simulink model "Example_1_Simu"  (R2023a)
settings: Solver=ode45  StartTime=0.0  StopTime=t_end  FixedStep=1e-6  RelTol=relTol  AbsTol=absTol
undefined symbols (not defined in the file or in its folder): Ag, gamma, InitialOffset, omegag, RayCoe, X, Y, Z
libraries: slrealtimeloglib x26, nesl_utility x19, sm_lib x9, OxDynamicsContact x4, sharedtransform x1
settings Model: Creator=sagat  LastModifiedBy=sagat
settings SolverCC: ConcurrentTasks=on
settings DataIOCC: Decimation=50  FinalStateName=xInitial  InitialState=xinitial  SaveOperatingPoint=on  SaveState=on  ReturnWorkspaceOutputs=off  LoggingToFile=on  LoggingFileName=D:\CODING\Simscape\FinalInvestigation\UniformDamping\LongBeam\ColumnResults
settings OptimizationCC: BlockReduction=off  DefaultParameterBehavior=Inlined  OptimizeBlockIOStorage=off  BufferReuse=off  OptimizeDataStoreBuffers=off  BusAssignmentInplaceUpdate=off
settings DebuggingCC: UnconnectedInputMsg=warning  UnconnectedOutputMsg=warning  UnconnectedLineMsg=warning  SFUnexpectedBacktrackingDiag=warning  SFNoUnconditionalDefaultTransitionDiag=warning
settings HardwareCC: TargetBitPerPointer=64  TargetBitPerSizeT=64  TargetBitPerPtrDiffT=64  TargetLongLongMode=on  TargetIntDivRoundTo=Zero  TargetEndianess=LittleEndian  TargetWordSize=64  TargetHWDeviceType=MATLAB Host  ProdEqTarget=off
settings ModelReferenceCC: EnableRefExpFcnMdlSchedulingChecks=on
settings RTWCC: Description=Rapid Simulation Target  SystemTargetFile=rsim.tlc  GenCodeOnly=on  TemplateMakefile=rsim_default_tmf  GenerateReport=on  BuildConfiguration=Debug  LaunchReport=on  DLArmComputeVersion=19.05
settings CodeAppCC: ForceParamTrailComments=on  MATLABSourceComments=on  EnableCustomComments=on
settings RSimTargetCC: TargetLangStandard=C99 (ISO)  OptimizeReductions=off
settings ExplorerConfigSet: SimMechanicsOpenEditorOnUpdate=off

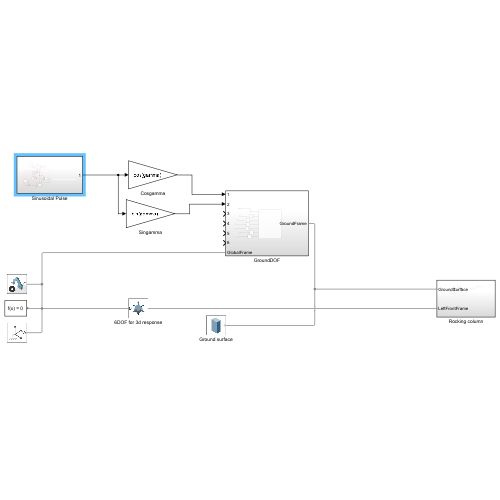
[thumbnail: Simulink's stored preview of the top-level diagram]
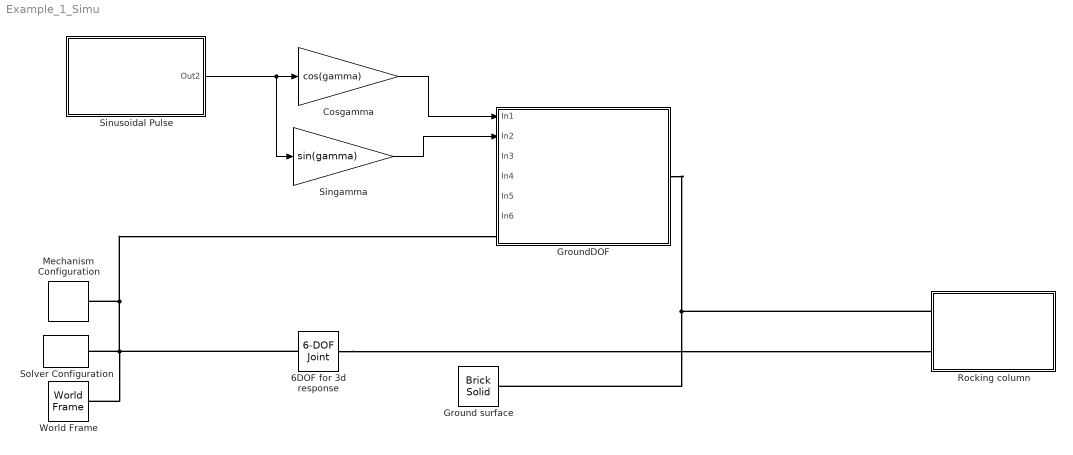
== system Example_1_Simu ==
  6DOF for 3d response : sm_lib/Joints/6-DOF Joint  JointMode=Normal  SenseConstraintForce=off  SenseConstraintForceX=off  SenseConstraintForceY=off  SenseConstraintForceZ=off  SenseConstraintTorque=off  SenseConstraintTorqueX=off  SenseConstraintTorqueY=off  SenseConstraintTorqueZ=off  SenseTotalForce=off  SenseTotalForceX=off  SenseTotalForceY=off  SenseTotalForceZ=off  SenseTotalTorque=off  SenseTotalTorqueX=off  SenseTotalTorqueY=off  SenseTotalTorqueZ=off  CompositeWrenchDir=FollowerOnBase  CompositeWrenchFrame=BaseFrame  PxEquilibriumPosition=0  PxEquilibriumPositionUnits=m  PxSpringStiffness=0  PxSpringStiffnessUnits=N/m  PxDampingCoefficient=0  PxDampingCoefficientUnits=N/(m/s)  PxTorqueActuationMode=NoTorque  PxMotionActuationMode=ComputedMotion  PxSensePosition=off  PxSenseVelocity=off  PxSenseAcceleration=off  PxSenseTorqueForce=off  PxSenseLowerLimitTorqueForce=off  PxSenseUpperLimitTorqueForce=off  PxLowerLimitSpecify=off  PxLowerLimitBound=-1  PxLowerLimitBoundUnits=m  PxLowerLimitStiffness=1e6  PxLowerLimitStiffnessUnits=N/m  PxLowerLimitDamping=1e3  PxLowerLimitDampingUnits=N/(m/s)  PxLowerLimitTransitionRegionWidth=1e-4  PxLowerLimitTransitionRegionWidthUnits=m  PxUpperLimitSpecify=off  PxUpperLimitBound=1  PxUpperLimitBoundUnits=m  PxUpperLimitStiffness=1e6  PxUpperLimitStiffnessUnits=N/m  PxUpperLimitDamping=1e3  PxUpperLimitDampingUnits=N/(m/s)  PxUpperLimitTransitionRegionWidth=1e-4  PxUpperLimitTransitionRegionWidthUnits=m  PxPositionTargetSpecify=on  PxPositionTargetPriority=High  PxPositionTargetValue=0  PxPositionTargetValueUnits=m  PxVelocityTargetSpecify=on  PxVelocityTargetPriority=High  PxVelocityTargetValue=0  PxVelocityTargetValueUnits=m/s  PyEquilibriumPosition=0  PyEquilibriumPositionUnits=m  PySpringStiffness=0  PySpringStiffnessUnits=N/m  PyDampingCoefficient=0  PyDampingCoefficientUnits=N/(m/s)  PyTorqueActuationMode=NoTorque  PyMotionActuationMode=ComputedMotion  PySensePosition=off  PySenseVelocity=off  PySenseAcceleration=off  PySenseTorqueForce=off  PySenseLowerLimitTorqueForce=off  PySenseUpperLimitTorqueForce=off  PyLowerLimitSpecify=off  PyLowerLimitBound=-1  PyLowerLimitBoundUnits=m  PyLowerLimitStiffness=1e6  PyLowerLimitStiffnessUnits=N/m  PyLowerLimitDamping=1e3  PyLowerLimitDampingUnits=N/(m/s)  PyLowerLimitTransitionRegionWidth=1e-4  PyLowerLimitTransitionRegionWidthUnits=m  PyUpperLimitSpecify=off  PyUpperLimitBound=1  PyUpperLimitBoundUnits=m  PyUpperLimitStiffness=1e6  PyUpperLimitStiffnessUnits=N/m  PyUpperLimitDamping=1e3  PyUpperLimitDampingUnits=N/(m/s)  PyUpperLimitTransitionRegionWidth=1e-4  PyUpperLimitTransitionRegionWidthUnits=m  PyPositionTargetSpecify=on  PyPositionTargetPriority=High  PyPositionTargetValue=0  PyPositionTargetValueUnits=m  PyVelocityTargetSpecify=on  PyVelocityTargetPriority=High  PyVelocityTargetValue=0  PyVelocityTargetValueUnits=m/s  PzEquilibriumPosition=0  PzEquilibriumPositionUnits=m  PzSpringStiffness=0  PzSpringStiffnessUnits=N/m  PzDampingCoefficient=0  PzDampingCoefficientUnits=N/(m/s)  PzTorqueActuationMode=NoTorque  PzMotionActuationMode=ComputedMotion  PzSensePosition=off  PzSenseVelocity=off  PzSenseAcceleration=off  PzSenseTorqueForce=off  PzSenseLowerLimitTorqueForce=off  PzSenseUpperLimitTorqueForce=off  PzLowerLimitSpecify=off  PzLowerLimitBound=-1  PzLowerLimitBoundUnits=m  PzLowerLimitStiffness=1e6  PzLowerLimitStiffnessUnits=N/m  PzLowerLimitDamping=1e3  PzLowerLimitDampingUnits=N/(m/s)  PzLowerLimitTransitionRegionWidth=1e-4  PzLowerLimitTransitionRegionWidthUnits=m  PzUpperLimitSpecify=off  PzUpperLimitBound=1  PzUpperLimitBoundUnits=m  PzUpperLimitStiffness=1e6  PzUpperLimitStiffnessUnits=N/m  PzUpperLimitDamping=1e3  PzUpperLimitDampingUnits=N/(m/s)  PzUpperLimitTransitionRegionWidth=1e-4  PzUpperLimitTransitionRegionWidthUnits=m  PzPositionTargetSpecify=on  PzPositionTargetPriority=High  PzPositionTargetValue=zc  PzPositionTargetValueUnits=m  PzVelocityTargetSpecify=on  PzVelocityTargetPriority=High  PzVelocityTargetValue=0  PzVelocityTargetValueUnits=m/s  SphEqPosRotationMethod=None  SphEqPosRotationAngleUnits=rad  SphEqPosRotationStandardAxis=-Y  SphEqPosRotationAngle=alphacg  SphEqPosRotationArbitraryAxis=[0 0 1]  SphEqPosFollAlignAxisA=+X  SphEqPosBaseAlignAxisA=+Y  SphEqPosFollAlignAxisB=+Y  SphEqPosBaseAlignAxisB=+Z  SphEqPosRotationSequenceAxes=FollowerAxes  SphEqPosRotationSequence=XYX  SphEqPosRotationSequenceAngles=[0 0 0]  SphEqPosRotationSequenceAnglesUnits=deg  SphEqPosRotationMatrix=[1 0 0; 0 1 0; 0 0 1]  SphEqPosQuaternion=[1 0 0 0]  SphSpringStiffness=0  SphSpringStiffnessUnits=N*m/rad  SphDampingCoefficient=0  SphDampingCoefficientUnits=N*m/(rad/s)  SphActuateTorqueX=off  SphActuateTorqueY=off  SphActuateTorqueZ=off  SphActuateTorque=off  SphTorqueActuationMode=NoTorque  SphMotionActuationMode=ComputedMotion  SphActuationFrame=BaseFrame  SphSensePosition=off  SphSenseVelocityX=off  SphSenseVelocityY=off  SphSenseVelocityZ=off  SphSenseVelocity=off  SphSenseAccelerationX=off  SphSenseAccelerationY=off  SphSenseAccelerationZ=off  SphSenseAcceleration=off  SphSenseTorqueX=off  SphSenseTorqueY=off  SphSenseTorqueZ=off  SphSenseTorqueForce=off  SphSenseLowerLimitTorqueMag=off  SphSenseUpperLimitTorqueMag=off  SphSensingFrame=BaseFrame  SphLowerLimitSpecify=off  SphLowerLimitBound=15  SphLowerLimitBoundUnits=deg  SphLowerLimitStiffness=1e4  SphLowerLimitStiffnessUnits=N*m/deg  SphLowerLimitDamping=10  SphLowerLimitDampingUnits=N*m/(deg/s)  SphLowerLimitTransitionRegionWidth=0.1  SphLowerLimitTransitionRegionWidthUnits=deg  SphUpperLimitSpecify=off  SphUpperLimitBound=45  SphUpperLimitBoundUnits=deg  SphUpperLimitStiffness=1e4  SphUpperLimitStiffnessUnits=N*m/deg  SphUpperLimitDamping=10  SphUpperLimitDampingUnits=N*m/(deg/s)  SphUpperLimitTransitionRegionWidth=0.1  SphUpperLimitTransitionRegionWidthUnits=deg  SphPositionTargetRotationMethod=StandardAxis  SphPositionTargetRotationAngleUnits=rad  SphPositionTargetRotationStandardAxis=-Y  SphPositionTargetRotationAngle=initialRotation  SphPositionTargetRotationArbitraryAxis=[0 0 1]  SphPositionTargetFollAlignAxisA=+X  SphPositionTargetBaseAlignAxisA=+Y  SphPositionTargetFollAlignAxisB=+Y  SphPositionTargetBaseAlignAxisB=+Z  SphPositionTargetRotationSequenceAxes=FollowerAxes  SphPositionTargetRotationSequence=XYX  SphPositionTargetRotationSequenceAngles=[0 0 0]  SphPositionTargetRotationSequenceAnglesUnits=deg  SphPositionTargetRotationMatrix=[1 0 0; 0 1 0; 0 0 1]  SphPositionTargetQuaternion=[1 0 0 0]  SphPositionTargetSpecify=on  SphPositionTargetPriority=High  SphVelocityTargetValue=[0 0 0]  SphVelocityTargetValueUnits=deg/s  SphVelocityTargetSpecify=on  SphVelocityTargetPriority=High  SphVelocityTargetInFollowerFrame=on
  Cosgamma : Gain  Gain=cos(gamma)
  Ground surface : sm_lib/Body Elements/Brick Solid  GraphicAmbientColor=[0.15 0.15 0.15 1.0]  BasedOnType=Density  BrickDimensions=[5 5 0.01]  BrickDimensionsUnits=m  CenterOfMass=[0 0 0]  CenterOfMassUnits=m  GraphicDiffuseColor=[0.5 0.5 0.5]  Density=1  DensityUnits=kg/m^3  DoExposeReferenceFrame=on  GraphicEmissiveColor=[0.0 0.0 0.0 1.0]  ExportEntireGeometry=off  SerializedFrames=<Frames/>  MarkerShape=Sphere  MarkerSize=10  GraphicType=FromGeometry  InertiaType=CalculateFromGeometry  Mass=1  MassUnits=kg  MomentsOfInertia=[1 1 1]  MomentsOfInertiaUnits=kg*m^2  GraphicOpacity=1.0  ProductsOfInertia=[0 0 0]  ProductsOfInertiaUnits=kg*m^2  GraphicShininess=75  GraphicSpecularColor=[0.5 0.5 0.5 1.0]  GraphicVisPropType=SimpleVisualProperties
  GroundDOF : Subsystem
  Mechanism Configuration : sm_lib/Utilities/Mechanism Configuration  UniformGravity=Constant  GravityVector=[0 0 -9.80665]  GravityVectorUnits=m/s^2  LinearizationDelta=0.001  JointModeTransitionNonlinearIterations=2
  Rocking column : Subsystem
  Singamma : Gain  Gain=sin(gamma)
  Sinusoidal Pulse : Subsystem
  Solver Configuration : nesl_utility/Solver Configuration  PhysicalDomain=network_engine_domain  SubClassName=solver  LeftPortType=input  RightPortType=generic  Tones=[]  Harmonics=[]  SimulateNoise=off  Profile=off  UseLocalSampling=off  EnableSwitchedLinearOptims=on  FrequencyDomain=off  UseCCode=off  RelTol=0.001  AbsTol=1e-06  MinStep=1e-09  ToWorkspace=off  RevertToSquareIcSolve=off  NumHomotopyIterations=100  PhasorMode=off  PhasorModeNumHarmonics=1  ConsistencySolver=NEWTON_FTOL  IndexReductionMethod=DerivativeReplacement  DoDC=off  ResidualTolerance=1e-09  ConsistencyTolSource=GLOBAL  ConsistencyAbsTol=0.001  ConsistencyRelTol=0.001  ConsistencyTolFactor=0.001  UseLocalSolver=off  LocalSolverChoice=NE_BACKWARD_EULER_ADVANCER  ResolveIndetEquations=on  FunctionEvalNumThread=1  LocalSolverSampleTime=0.001  DoFixedCost=off  MaxNonlinIter=3  MaxModeIter=2  ComputeImpulses=off  ImpulseIterations=2  LinearAlgebra=auto  LinearAlgebraNumThread=0  EquationFormulation=NE_TIME_EF  DelaysMemoryBudget=1024  AutomaticFiltering=on  FilteringTimeConstant=0.001  PartitionStorageMethod=AS_NEEDED  PartitionMemoryBudget=1024  PartitionMethod=ROBUST
  World Frame : sm_lib/Frames and Transforms/World Frame
  wires:
  Cosgamma/1 -> GroundDOF/1(In1)
  Sinusoidal Pulse/1(Out2) -> Singamma/1, Cosgamma/1
  Singamma/1 -> GroundDOF/2(In2)
  connections:
  World Frame/RConn1 -- GroundDOF/LConn1 -- Mechanism Configuration/RConn1 -- 6DOF for 3d response/LConn1 -- Solver Configuration/RConn1
  6DOF for 3d response/RConn1 -- Rocking column/LConn2
  GroundDOF/RConn1 -- Rocking column/LConn1 -- Ground surface/RConn1

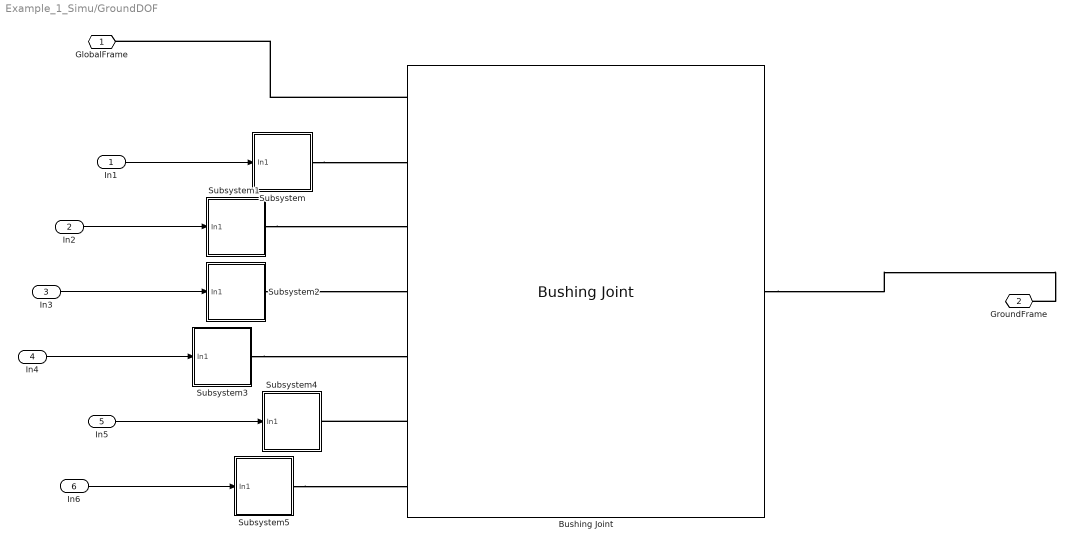
== system Example_1_Simu/GroundDOF ==
  In1 : Inport
  In2 : Inport  Port=2
  In3 : Inport  Port=3
  In4 : Inport  Port=4
  In5 : Inport  Port=5
  In6 : Inport  Port=6
  Bushing Joint : sm_lib/Joints/Bushing Joint  JointMode=Normal  SenseConstraintForce=off  SenseConstraintForceX=off  SenseConstraintForceY=off  SenseConstraintForceZ=off  SenseConstraintTorque=off  SenseConstraintTorqueX=off  SenseConstraintTorqueY=off  SenseConstraintTorqueZ=off  SenseTotalForce=off  SenseTotalForceX=off  SenseTotalForceY=off  SenseTotalForceZ=off  SenseTotalTorque=off  SenseTotalTorqueX=off  SenseTotalTorqueY=off  SenseTotalTorqueZ=off  CompositeWrenchDir=FollowerOnBase  CompositeWrenchFrame=BaseFrame  PxEquilibriumPosition=0  PxEquilibriumPositionUnits=m  PxSpringStiffness=0  PxSpringStiffnessUnits=N/m  PxDampingCoefficient=0  PxDampingCoefficientUnits=N/(m/s)  PxTorqueActuationMode=ComputedTorque  PxMotionActuationMode=InputMotion  PxSensePosition=off  PxSenseVelocity=off  PxSenseAcceleration=off  PxSenseTorqueForce=off  PxSenseLowerLimitTorqueForce=off  PxSenseUpperLimitTorqueForce=off  PxLowerLimitSpecify=off  PxLowerLimitBound=-1  PxLowerLimitBoundUnits=m  PxLowerLimitStiffness=1e6  PxLowerLimitStiffnessUnits=N/m  PxLowerLimitDamping=1e3  PxLowerLimitDampingUnits=N/(m/s)  PxLowerLimitTransitionRegionWidth=1e-4  PxLowerLimitTransitionRegionWidthUnits=m  PxUpperLimitSpecify=off  PxUpperLimitBound=1  PxUpperLimitBoundUnits=m  PxUpperLimitStiffness=1e6  PxUpperLimitStiffnessUnits=N/m  PxUpperLimitDamping=1e3  PxUpperLimitDampingUnits=N/(m/s)  PxUpperLimitTransitionRegionWidth=1e-4  PxUpperLimitTransitionRegionWidthUnits=m  PxPositionTargetSpecify=off  PxPositionTargetPriority=High  PxPositionTargetValue=0  PxPositionTargetValueUnits=m  PxVelocityTargetSpecify=off  PxVelocityTargetPriority=High  PxVelocityTargetValue=0  PxVelocityTargetValueUnits=m/s  PyEquilibriumPosition=0  PyEquilibriumPositionUnits=m  PySpringStiffness=0  PySpringStiffnessUnits=N/m  PyDampingCoefficient=0  PyDampingCoefficientUnits=N/(m/s)  PyTorqueActuationMode=ComputedTorque  PyMotionActuationMode=InputMotion  PySensePosition=off  PySenseVelocity=off  PySenseAcceleration=off  PySenseTorqueForce=off  PySenseLowerLimitTorqueForce=off  PySenseUpperLimitTorqueForce=off  PyLowerLimitSpecify=off  PyLowerLimitBound=-1  PyLowerLimitBoundUnits=m  PyLowerLimitStiffness=1e6  PyLowerLimitStiffnessUnits=N/m  PyLowerLimitDamping=1e3  PyLowerLimitDampingUnits=N/(m/s)  PyLowerLimitTransitionRegionWidth=1e-4  PyLowerLimitTransitionRegionWidthUnits=m  PyUpperLimitSpecify=off  PyUpperLimitBound=1  PyUpperLimitBoundUnits=m  PyUpperLimitStiffness=1e6  PyUpperLimitStiffnessUnits=N/m  PyUpperLimitDamping=1e3  PyUpperLimitDampingUnits=N/(m/s)  PyUpperLimitTransitionRegionWidth=1e-4  PyUpperLimitTransitionRegionWidthUnits=m  PyPositionTargetSpecify=off  PyPositionTargetPriority=High  PyPositionTargetValue=0  PyPositionTargetValueUnits=m  PyVelocityTargetSpecify=off  PyVelocityTargetPriority=High  PyVelocityTargetValue=0  PyVelocityTargetValueUnits=m/s  PzEquilibriumPosition=0  PzEquilibriumPositionUnits=m  PzSpringStiffness=0  PzSpringStiffnessUnits=N/m  PzDampingCoefficient=0  PzDampingCoefficientUnits=N/(m/s)  PzTorqueActuationMode=ComputedTorque  PzMotionActuationMode=InputMotion  PzSensePosition=off  PzSenseVelocity=off  PzSenseAcceleration=off  PzSenseTorqueForce=off  PzSenseLowerLimitTorqueForce=off  PzSenseUpperLimitTorqueForce=off  PzLowerLimitSpecify=off  PzLowerLimitBound=-1  PzLowerLimitBoundUnits=m  PzLowerLimitStiffness=1e6  PzLowerLimitStiffnessUnits=N/m  PzLowerLimitDamping=1e3  PzLowerLimitDampingUnits=N/(m/s)  PzLowerLimitTransitionRegionWidth=1e-4  PzLowerLimitTransitionRegionWidthUnits=m  PzUpperLimitSpecify=off  PzUpperLimitBound=1  PzUpperLimitBoundUnits=m  PzUpperLimitStiffness=1e6  PzUpperLimitStiffnessUnits=N/m  PzUpperLimitDamping=1e3  PzUpperLimitDampingUnits=N/(m/s)  PzUpperLimitTransitionRegionWidth=1e-4  PzUpperLimitTransitionRegionWidthUnits=m  PzPositionTargetSpecify=off  PzPositionTargetPriority=High  PzPositionTargetValue=0  PzPositionTargetValueUnits=m  PzVelocityTargetSpecify=off  PzVelocityTargetPriority=High  PzVelocityTargetValue=0  PzVelocityTargetValueUnits=m/s  RxEquilibriumPosition=0  RxEquilibriumPositionUnits=deg  RxSpringStiffness=0  RxSpringStiffnessUnits=N*m/deg  RxDampingCoefficient=0  RxDampingCoefficientUnits=N*m/(deg/s)  RxTorqueActuationMode=ComputedTorque  RxMotionActuationMode=InputMotion  RxSensePosition=off  RxSenseVelocity=off  RxSenseAcceleration=off  RxSenseTorqueForce=off  RxSenseLowerLimitTorqueForce=off  RxSenseUpperLimitTorqueForce=off  RxLowerLimitSpecify=off  RxLowerLimitBound=-90  RxLowerLimitBoundUnits=deg  RxLowerLimitStiffness=1e4  RxLowerLimitStiffnessUnits=N*m/deg  RxLowerLimitDamping=10  RxLowerLimitDampingUnits=N*m/(deg/s)  RxLowerLimitTransitionRegionWidth=0.1  RxLowerLimitTransitionRegionWidthUnits=deg  RxUpperLimitSpecify=off  RxUpperLimitBound=90  RxUpperLimitBoundUnits=deg  RxUpperLimitStiffness=1e4  RxUpperLimitStiffnessUnits=N*m/deg  RxUpperLimitDamping=10  RxUpperLimitDampingUnits=N*m/(deg/s)  RxUpperLimitTransitionRegionWidth=0.1  RxUpperLimitTransitionRegionWidthUnits=deg  RxPositionTargetSpecify=off  RxPositionTargetPriority=High  RxPositionTargetValue=0  RxPositionTargetValueUnits=deg  RxVelocityTargetSpecify=off  RxVelocityTargetPriority=High  RxVelocityTargetValue=0  RxVelocityTargetValueUnits=deg/s  RyEquilibriumPosition=0  RyEquilibriumPositionUnits=deg  RySpringStiffness=0  RySpringStiffnessUnits=N*m/deg  RyDampingCoefficient=0  RyDampingCoefficientUnits=N*m/(deg/s)  RyTorqueActuationMode=ComputedTorque  RyMotionActuationMode=InputMotion  RySensePosition=off  RySenseVelocity=off  RySenseAcceleration=off  RySenseTorqueForce=off  RySenseLowerLimitTorqueForce=off  RySenseUpperLimitTorqueForce=off  RyLowerLimitSpecify=off  RyLowerLimitBound=-90  RyLowerLimitBoundUnits=deg  RyLowerLimitStiffness=1e4  RyLowerLimitStiffnessUnits=N*m/deg  RyLowerLimitDamping=10  RyLowerLimitDampingUnits=N*m/(deg/s)  RyLowerLimitTransitionRegionWidth=0.1  RyLowerLimitTransitionRegionWidthUnits=deg  RyUpperLimitSpecify=off  RyUpperLimitBound=90  RyUpperLimitBoundUnits=deg  RyUpperLimitStiffness=1e4  RyUpperLimitStiffnessUnits=N*m/deg  RyUpperLimitDamping=10  RyUpperLimitDampingUnits=N*m/(deg/s)  RyUpperLimitTransitionRegionWidth=0.1  RyUpperLimitTransitionRegionWidthUnits=deg  RyPositionTargetSpecify=off  RyPositionTargetPriority=High  RyPositionTargetValue=0  RyPositionTargetValueUnits=deg  RyVelocityTargetSpecify=off  RyVelocityTargetPriority=High  RyVelocityTargetValue=0  RyVelocityTargetValueUnits=deg/s  RzEquilibriumPosition=0  RzEquilibriumPositionUnits=deg  RzSpringStiffness=0  RzSpringStiffnessUnits=N*m/deg  RzDampingCoefficient=0  RzDampingCoefficientUnits=N*m/(deg/s)  RzTorqueActuationMode=ComputedTorque  RzMotionActuationMode=InputMotion  RzSensePosition=off  RzSenseVelocity=off  RzSenseAcceleration=off  RzSenseTorqueForce=off  RzSenseLowerLimitTorqueForce=off  RzSenseUpperLimitTorqueForce=off  RzLowerLimitSpecify=off  RzLowerLimitBound=-90  RzLowerLimitBoundUnits=deg  RzLowerLimitStiffness=1e4  RzLowerLimitStiffnessUnits=N*m/deg  RzLowerLimitDamping=10  RzLowerLimitDampingUnits=N*m/(deg/s)  RzLowerLimitTransitionRegionWidth=0.1  RzLowerLimitTransitionRegionWidthUnits=deg  RzUpperLimitSpecify=off  RzUpperLimitBound=90  RzUpperLimitBoundUnits=deg  RzUpperLimitStiffness=1e4  RzUpperLimitStiffnessUnits=N*m/deg  RzUpperLimitDamping=10  RzUpperLimitDampingUnits=N*m/(deg/s)  RzUpperLimitTransitionRegionWidth=0.1  RzUpperLimitTransitionRegionWidthUnits=deg  RzPositionTargetSpecify=off  RzPositionTargetPriority=High  RzPositionTargetValue=0  RzPositionTargetValueUnits=deg  RzVelocityTargetSpecify=off  RzVelocityTargetPriority=High  RzVelocityTargetValue=0  RzVelocityTargetValueUnits=deg/s
  Subsystem : Subsystem
  Subsystem1 : Subsystem
  Subsystem2 : Subsystem
  Subsystem3 : Subsystem
  Subsystem4 : Subsystem
  Subsystem5 : Subsystem
  GlobalFrame : PMIOPort  Side=Left
  GroundFrame : PMIOPort  Port=2  Side=Right
  wires:
  In1/1 -> Subsystem/1(In1)
  In5/1 -> Subsystem4/1(In1)
  In2/1 -> Subsystem1/1(In1)
  In3/1 -> Subsystem2/1(In1)
  In4/1 -> Subsystem3/1(In1)
  In6/1 -> Subsystem5/1(In1)
  connections:
  Bushing Joint/LConn1 -- GlobalFrame/RConn1
  Subsystem3/RConn1 -- Bushing Joint/LConn5
  Subsystem/RConn1 -- Bushing Joint/LConn2
  Bushing Joint/LConn6 -- Subsystem4/RConn1
  Subsystem2/RConn1 -- Bushing Joint/LConn4
  Subsystem5/RConn1 -- Bushing Joint/LConn7
  Bushing Joint/RConn1 -- GroundFrame/RConn1
  Subsystem1/RConn1 -- Bushing Joint/LConn3

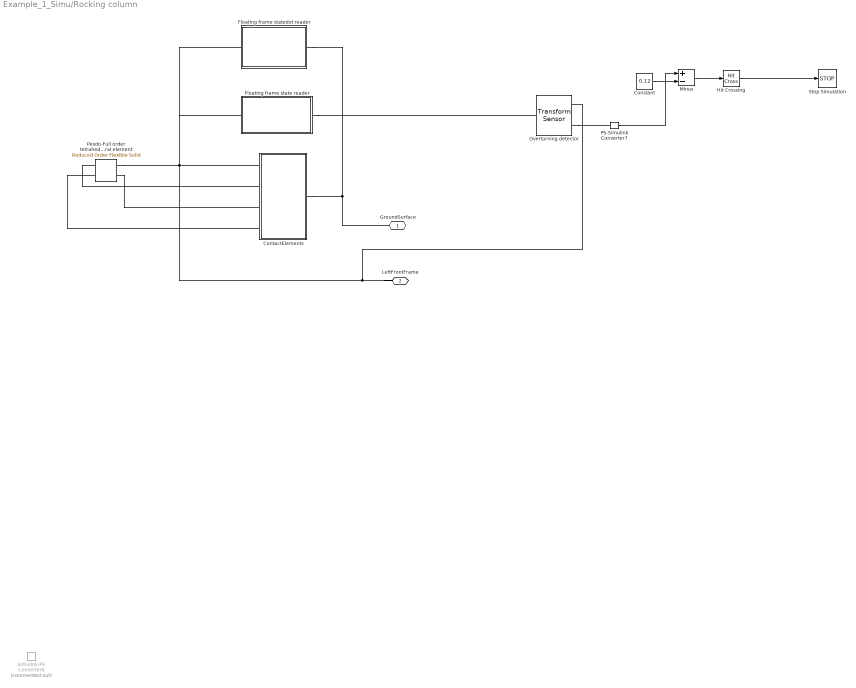
== system Example_1_Simu/Rocking column ==
  Constant : Constant  Value=0.12
  ContactElements : Subsystem
  Floating frame state reader : Subsystem
  Floating frame statedot reader : Subsystem
  Hit Crossing : HitCross
  Minus : Sum  Inputs=+-
  Overturning detector : sm_lib/Frames and Transforms/Transform Sensor  MeasurementFrame=Base  RotationSequence=XYX  SenseAngle=on  SenseAxis=off  SenseQ=off  SenseR=off  SenseRotationSequence=off  SenseOmegaX=off  SenseOmegaY=off  SenseOmegaZ=off  SenseQDot=off  SenseRDot=off  SenseRotationSequenceDot=off  SenseAlphaX=off  SenseAlphaY=off  SenseAlphaZ=off  SenseQDDot=off  SenseRDDot=off  SenseX=off  SenseY=off  SenseZ=off  SenseRad=off  SenseAzim=off  SenseDist=off  SenseInc=off  SenseXDot=off  SenseYDot=off  SenseZDot=off  SenseRadDot=off  SenseAzimDot=off  SenseDistDot=off  SenseIncDot=off  SenseXDDot=off  SenseYDDot=off  SenseZDDot=off  SenseRadDDot=off  SenseAzimDDot=off  SenseDistDDot=off  SenseIncDDot=off
  PS-Simulink Converter7 : nesl_utility/PS-Simulink Converter  PhysicalDomain=network_engine_domain  SubClassName=ps_output  LeftPortType=input  RightPortType=output  PseudoPeriodic=off  Frequencies=[]  VectorFormat=1-D array  Unit=inherit  AffineConversion=off
  Pesdo-Full order tetrahedral element : sm_lib/Body Elements/Flexible Bodies/Reduced Order Flexible Solid  GraphicAmbientColor=[0.15 0.15 0.15 1.0]  GraphicDiffuseColor=[0.5 0.5 0.5]  DampingType=DampingMatrix  GraphicEmissiveColor=[0.0 0.0 0.0 1.0]  GraphicFacetVertexIndices=[]  GeomFileName=D:\CODING\Simscape\ReducedSuperStructure&AxialDeformationInvestigation\WaterTank\Trial2.stl  InterfaceFrameOrientations=[1 0 0 0;1 0 0 0;1 0 0 0;1 0 0 0]  GraphicType=None  MassMatrix=Reduced.M  NumRetainedModes=1  NumberOfInterfaceFrames=4  GraphicOpacity=1.0  GraphicReconstructionMatrix=[]  ReductionType=None  InterfaceFrameOrigins=Reduced.P  GraphicShininess=75  GraphicSpecularColor=[0.5 0.5 0.5 1.0]  StiffnessMatrix=Reduced.K  GeomUnitType=FromUnitSystem  GraphicVertexCoordinates=[]  VisRecursionLimit=3  GraphicVisPropType=SimpleVisualProperties  LengthUnit=m  MassUnit=kg  TimeUnit=s  UnitSystemType=SI  ProportionalDampingAlpha=0  ProportionalDampingBeta=RayCoe(2)  UniformModalDampingRatio=0.05  DampingMatrix=Reduced.C
  Simulink-PS Converter6 : nesl_utility/Simulink-PS Converter  Commented=on  PhysicalDomain=network_engine_domain  SubClassName=ps_input  LeftPortType=input  RightPortType=output  PseudoPeriodic=off  Frequencies=[]  NoiseDistribution=none  NoiseParameters=[]  Unit=1  AffineConversion=off  FilteringAndDerivatives=provide  SimscapeFilterOrder=1  InputFilterTimeConstant=0.001  UdotUserProvided=0
  Stop Simulation : Stop
  GroundSurface : PMIOPort  Side=Left
  LeftFrontFrame : PMIOPort  Port=2  Side=Left
  wires:
  PS-Simulink Converter7/1 -> Minus/1
  Minus/1 -> Hit Crossing/1
  Hit Crossing/1 -> Stop Simulation/1
  Constant/1 -> Minus/2
  connections:
  Pesdo-Full order tetrahedral element/LConn1 -- Floating frame state reader/RConn1 -- Floating frame statedot reader/RConn1 -- ContactElements/LConn1 -- Overturning detector/RConn1 -- LeftFrontFrame/RConn1
  Pesdo-Full order tetrahedral element/RConn1 -- ContactElements/LConn2
  Pesdo-Full order tetrahedral element/LConn2 -- ContactElements/LConn3
  Pesdo-Full order tetrahedral element/RConn2 -- ContactElements/LConn4
  ContactElements/RConn1 -- Floating frame statedot reader/LConn1 -- Floating frame state reader/LConn1 -- Overturning detector/LConn1 -- GroundSurface/RConn1
  Overturning detector/RConn2 -- PS-Simulink Converter7/LConn1

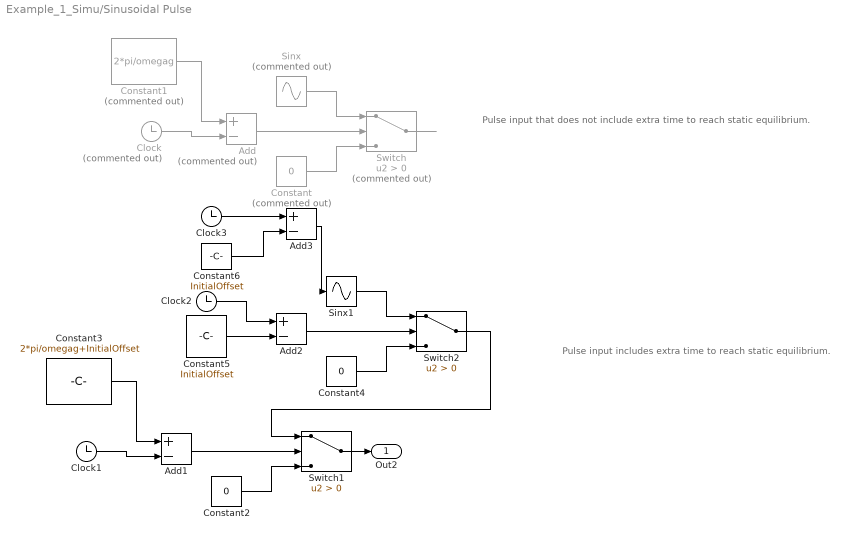
== system Example_1_Simu/Sinusoidal Pulse ==
  note: Pulse input that does not include extra time to reach static equilibrium.
  note: Pulse input includes extra time to reach static equilibrium.
  Add : Sum  Commented=on  Inputs=+-
  Add1 : Sum  Inputs=+-
  Add2 : Sum  Inputs=+-
  Add3 : Sum  Inputs=+-
  Clock : Clock  Commented=on
  Clock1 : Clock
  Clock2 : Clock
  Clock3 : Clock
  Constant : Constant  Commented=on  Value=0
  Constant1 : Constant  Commented=on  Value=2*pi/omegag
  Constant2 : Constant  Value=0
  Constant3 : Constant  Value=2*pi/omegag+InitialOffset
  Constant4 : Constant  Value=0
  Constant5 : Constant  Value=InitialOffset
  Constant6 : Constant  Value=InitialOffset
  Sinx : Sin  Commented=on  Amplitude=Ag  Frequency=omegag  SampleTime=0
  Sinx1 : Sin  TimeSource=Use external signal  Amplitude=Ag  Frequency=omegag  SampleTime=0
  Switch : Switch  Commented=on  Criteria=u2 > Threshold  SaturateOnIntegerOverflow=off  InputSameDT=off
  Switch1 : Switch  Criteria=u2 > Threshold  SaturateOnIntegerOverflow=off  InputSameDT=off
  Switch2 : Switch  Criteria=u2 > Threshold  SaturateOnIntegerOverflow=off  InputSameDT=off
  Out2 : Outport
  wires:
  Clock/1 -> Add/2
  Switch/1 -> ?
  Constant1/1 -> Add/1
  Sinx/1 -> Switch/1
  Constant/1 -> Switch/3
  Add/1 -> Switch/2
  Switch1/1 -> Out2/1
  Clock1/1 -> Add1/2
  Constant2/1 -> Switch1/3
  Add1/1 -> Switch1/2
  Constant3/1 -> Add1/1
  Switch2/1 -> Switch1/1
  Constant4/1 -> Switch2/3
  Add2/1 -> Switch2/2
  Sinx1/1 -> Switch2/1
  Clock2/1 -> Add2/1
  Constant5/1 -> Add2/2
  Clock3/1 -> Add3/1
  Constant6/1 -> Add3/2
  Add3/1 -> Sinx1/1

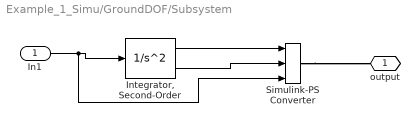
== system Example_1_Simu/GroundDOF/Subsystem ==
  In1 : Inport
  "Integrator, Second-Order" : SecondOrderIntegrator
  Simulink-PS Converter : nesl_utility/Simulink-PS Converter  PhysicalDomain=network_engine_domain  SubClassName=ps_input  LeftPortType=input  RightPortType=output  PseudoPeriodic=off  Frequencies=[]  NoiseDistribution=none  NoiseParameters=[]  Unit=1  AffineConversion=off  FilteringAndDerivatives=provide  SimscapeFilterOrder=1  InputFilterTimeConstant=0.001  UdotUserProvided=2
  output : PMIOPort  Side=Right
  wires:
  "Integrator, Second-Order"/1 -> Simulink-PS Converter/1
  "Integrator, Second-Order"/2 -> Simulink-PS Converter/2
  In1/1 -> "Integrator, Second-Order"/1, Simulink-PS Converter/3
  connections:
  Simulink-PS Converter/RConn1 -- output/RConn1

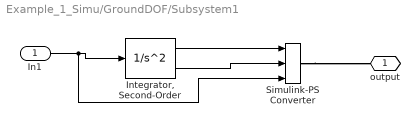
== system Example_1_Simu/GroundDOF/Subsystem1 ==
  In1 : Inport
  "Integrator, Second-Order" : SecondOrderIntegrator
  Simulink-PS Converter : nesl_utility/Simulink-PS Converter  PhysicalDomain=network_engine_domain  SubClassName=ps_input  LeftPortType=input  RightPortType=output  PseudoPeriodic=off  Frequencies=[]  NoiseDistribution=none  NoiseParameters=[]  Unit=1  AffineConversion=off  FilteringAndDerivatives=provide  SimscapeFilterOrder=1  InputFilterTimeConstant=0.001  UdotUserProvided=2
  output : PMIOPort  Side=Right
  wires:
  "Integrator, Second-Order"/1 -> Simulink-PS Converter/1
  "Integrator, Second-Order"/2 -> Simulink-PS Converter/2
  In1/1 -> "Integrator, Second-Order"/1, Simulink-PS Converter/3
  connections:
  Simulink-PS Converter/RConn1 -- output/RConn1

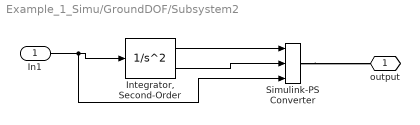
== system Example_1_Simu/GroundDOF/Subsystem2 ==
  In1 : Inport
  "Integrator, Second-Order" : SecondOrderIntegrator
  Simulink-PS Converter : nesl_utility/Simulink-PS Converter  PhysicalDomain=network_engine_domain  SubClassName=ps_input  LeftPortType=input  RightPortType=output  PseudoPeriodic=off  Frequencies=[]  NoiseDistribution=none  NoiseParameters=[]  Unit=1  AffineConversion=off  FilteringAndDerivatives=provide  SimscapeFilterOrder=1  InputFilterTimeConstant=0.001  UdotUserProvided=2
  output : PMIOPort  Side=Right
  wires:
  "Integrator, Second-Order"/1 -> Simulink-PS Converter/1
  "Integrator, Second-Order"/2 -> Simulink-PS Converter/2
  In1/1 -> "Integrator, Second-Order"/1, Simulink-PS Converter/3
  connections:
  Simulink-PS Converter/RConn1 -- output/RConn1

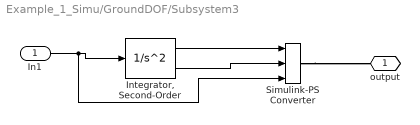
== system Example_1_Simu/GroundDOF/Subsystem3 ==
  In1 : Inport
  "Integrator, Second-Order" : SecondOrderIntegrator
  Simulink-PS Converter : nesl_utility/Simulink-PS Converter  PhysicalDomain=network_engine_domain  SubClassName=ps_input  LeftPortType=input  RightPortType=output  PseudoPeriodic=off  Frequencies=[]  NoiseDistribution=none  NoiseParameters=[]  Unit=1  AffineConversion=off  FilteringAndDerivatives=provide  SimscapeFilterOrder=1  InputFilterTimeConstant=0.001  UdotUserProvided=2
  output : PMIOPort  Side=Right
  wires:
  In1/1 -> Simulink-PS Converter/3, "Integrator, Second-Order"/1
  "Integrator, Second-Order"/2 -> Simulink-PS Converter/2
  "Integrator, Second-Order"/1 -> Simulink-PS Converter/1
  connections:
  Simulink-PS Converter/RConn1 -- output/RConn1

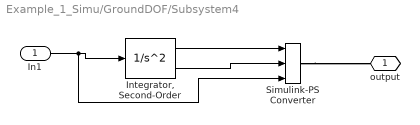
== system Example_1_Simu/GroundDOF/Subsystem4 ==
  In1 : Inport
  "Integrator, Second-Order" : SecondOrderIntegrator
  Simulink-PS Converter : nesl_utility/Simulink-PS Converter  PhysicalDomain=network_engine_domain  SubClassName=ps_input  LeftPortType=input  RightPortType=output  PseudoPeriodic=off  Frequencies=[]  NoiseDistribution=none  NoiseParameters=[]  Unit=1  AffineConversion=off  FilteringAndDerivatives=provide  SimscapeFilterOrder=1  InputFilterTimeConstant=0.001  UdotUserProvided=2
  output : PMIOPort  Side=Right
  wires:
  "Integrator, Second-Order"/1 -> Simulink-PS Converter/1
  "Integrator, Second-Order"/2 -> Simulink-PS Converter/2
  In1/1 -> "Integrator, Second-Order"/1, Simulink-PS Converter/3
  connections:
  Simulink-PS Converter/RConn1 -- output/RConn1

== system Example_1_Simu/GroundDOF/Subsystem5 ==
  In1 : Inport
  "Integrator, Second-Order" : SecondOrderIntegrator
  Simulink-PS Converter : nesl_utility/Simulink-PS Converter  PhysicalDomain=network_engine_domain  SubClassName=ps_input  LeftPortType=input  RightPortType=output  PseudoPeriodic=off  Frequencies=[]  NoiseDistribution=none  NoiseParameters=[]  Unit=1  AffineConversion=off  FilteringAndDerivatives=provide  SimscapeFilterOrder=1  InputFilterTimeConstant=0.001  UdotUserProvided=2
  output : PMIOPort  Side=Right
  wires:
  "Integrator, Second-Order"/1 -> Simulink-PS Converter/1
  "Integrator, Second-Order"/2 -> Simulink-PS Converter/2
  In1/1 -> "Integrator, Second-Order"/1, Simulink-PS Converter/3
  connections:
  Simulink-PS Converter/RConn1 -- output/RConn1

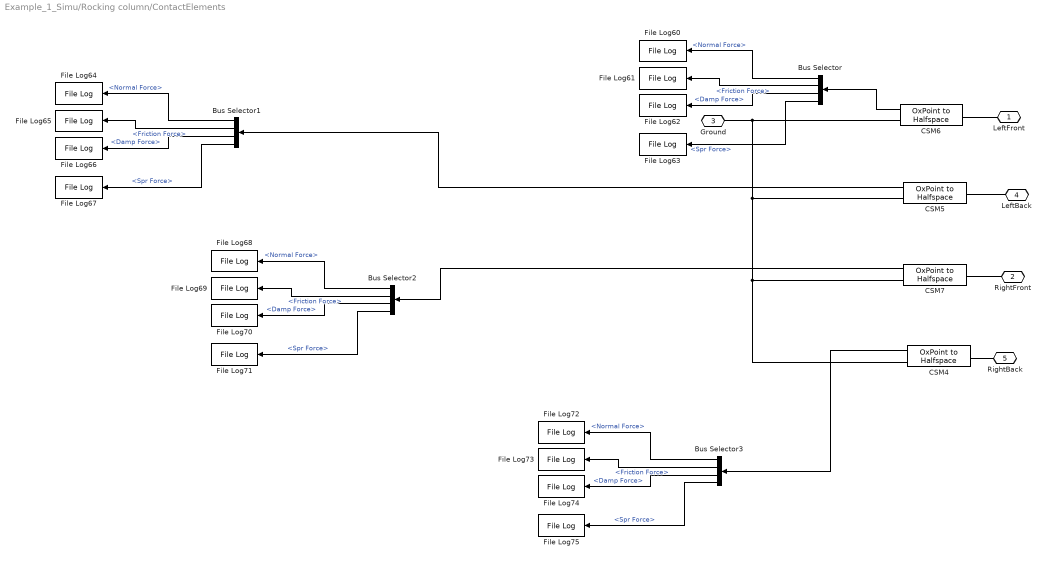
== system Example_1_Simu/Rocking column/ContactElements ==
  Bus Selector{,1..3} (4 alike) : BusSelector  OutputSignals=Normal Force,Friction Force,Damp Force,Spr Force
  CSM{4..7} (4 alike) : OxDynamicsContact/OxPoint to Halfspace  plane_lenx=40  plane_leny=40  force_law=Oxford Linear  k_contact=kk2  b_contact=cc1  pen_full_damp_F=1e-4  pen_exponent=1  custom_param_1=1  custom_param_2=1  friction_law=Oxford Friction  mu_kinetic=0.5  mu_static=muf  v_thr=0.001  k_f=k_n  c_f=c_n  vis_on=off  vis_opc_en=0  vis_len_plaBz=0.005  vis_clr=[0.9 0.2 0.2]  vis_opc=0.7
  File Log{60..75} (16 alike) : slrealtimeloglib/File Log  decimation=200  inputProcessing=Elements as channels (sample based)
  LeftFront : PMIOPort  Side=Left
  RightFront : PMIOPort  Port=2  Side=Left
  Ground : PMIOPort  Port=3  Side=Right
  LeftBack : PMIOPort  Port=4  Side=Left
  RightBack : PMIOPort  Port=5  Side=Left
  wires:
  CSM4/1 -> Bus Selector3/1
  CSM6/1 -> Bus Selector/1
  Bus Selector/1 -> File Log60/1  "<Normal Force>"
  Bus Selector/2 -> File Log61/1  "<Friction Force>"
  Bus Selector/3 -> File Log62/1  "<Damp Force>"
  Bus Selector/4 -> File Log63/1  "<Spr Force>"
  Bus Selector1/3 -> File Log66/1  "<Damp Force>"
  Bus Selector1/4 -> File Log67/1  "<Spr Force>"
  Bus Selector1/1 -> File Log64/1  "<Normal Force>"
  Bus Selector1/2 -> File Log65/1  "<Friction Force>"
  Bus Selector2/4 -> File Log71/1  "<Spr Force>"
  Bus Selector2/3 -> File Log70/1  "<Damp Force>"
  CSM7/1 -> Bus Selector2/1
  Bus Selector2/1 -> File Log68/1  "<Normal Force>"
  Bus Selector2/2 -> File Log69/1  "<Friction Force>"
  Bus Selector3/4 -> File Log75/1  "<Spr Force>"
  Bus Selector3/3 -> File Log74/1  "<Damp Force>"
  Bus Selector3/1 -> File Log72/1  "<Normal Force>"
  Bus Selector3/2 -> File Log73/1  "<Friction Force>"
  CSM5/1 -> Bus Selector1/1
  connections:
  CSM7/LConn1 -- RightFront/RConn1
  CSM6/RConn1 -- CSM4/RConn1 -- CSM7/RConn1 -- CSM5/RConn1 -- Ground/RConn1
  CSM4/LConn1 -- RightBack/RConn1
  CSM5/LConn1 -- LeftBack/RConn1
  CSM6/LConn1 -- LeftFront/RConn1

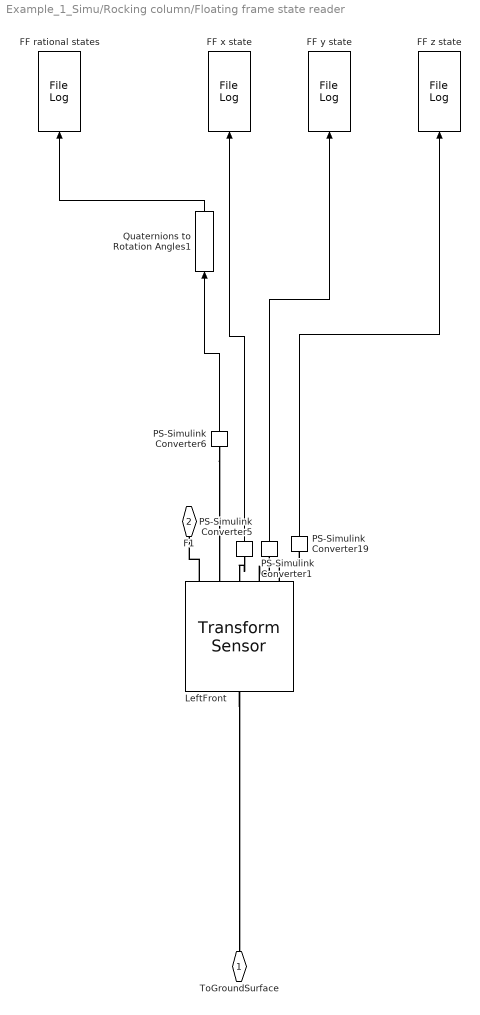
== system Example_1_Simu/Rocking column/Floating frame state reader ==
  " LeftFront" : sm_lib/Frames and Transforms/Transform Sensor  MeasurementFrame=Base  RotationSequence=XYX  SenseAngle=off  SenseAxis=off  SenseQ=on  SenseR=off  SenseRotationSequence=off  SenseOmegaX=off  SenseOmegaY=off  SenseOmegaZ=off  SenseQDot=off  SenseRDot=off  SenseRotationSequenceDot=off  SenseAlphaX=off  SenseAlphaY=off  SenseAlphaZ=off  SenseQDDot=off  SenseRDDot=off  SenseX=on  SenseY=on  SenseZ=on  SenseRad=off  SenseAzim=off  SenseDist=off  SenseInc=off  SenseXDot=off  SenseYDot=off  SenseZDot=off  SenseRadDot=off  SenseAzimDot=off  SenseDistDot=off  SenseIncDot=off  SenseXDDot=off  SenseYDDot=off  SenseZDDot=off  SenseRadDDot=off  SenseAzimDDot=off  SenseDistDDot=off  SenseIncDDot=off
  FF rational states : slrealtimeloglib/File Log  decimation=200  inputProcessing=Elements as channels (sample based)
  FF x state : slrealtimeloglib/File Log  decimation=200  inputProcessing=Elements as channels (sample based)
  FF y state : slrealtimeloglib/File Log  decimation=200  inputProcessing=Elements as channels (sample based)
  FF z state : slrealtimeloglib/File Log  decimation=200  inputProcessing=Elements as channels (sample based)
  PS-Simulink Converter{1,5..6,19} (4 alike) : nesl_utility/PS-Simulink Converter  PhysicalDomain=network_engine_domain  SubClassName=ps_output  LeftPortType=input  RightPortType=output  PseudoPeriodic=off  Frequencies=[]  VectorFormat=1-D array  Unit=inherit  AffineConversion=off
  Quaternions to Rotation Angles1 : sharedtransform/Quaternions to Rotation Angles  rotationOrder=XYZ  aMode=aMode
  ToGroundSurface : PMIOPort  Side=Left
  F1 : PMIOPort  Port=2  Side=Right
  wires:
  PS-Simulink Converter6/1 -> Quaternions to Rotation Angles1/1
  PS-Simulink Converter1/1 -> FF y state/1
  Quaternions to Rotation Angles1/1 -> FF rational states/1
  PS-Simulink Converter5/1 -> FF x state/1
  PS-Simulink Converter19/1 -> FF z state/1
  connections:
  " LeftFront"/RConn1 -- F1/RConn1
  PS-Simulink Converter6/LConn1 -- " LeftFront"/RConn2
  PS-Simulink Converter5/LConn1 -- " LeftFront"/RConn3
  " LeftFront"/RConn4 -- PS-Simulink Converter1/LConn1
  " LeftFront"/LConn1 -- ToGroundSurface/RConn1
  " LeftFront"/RConn5 -- PS-Simulink Converter19/LConn1

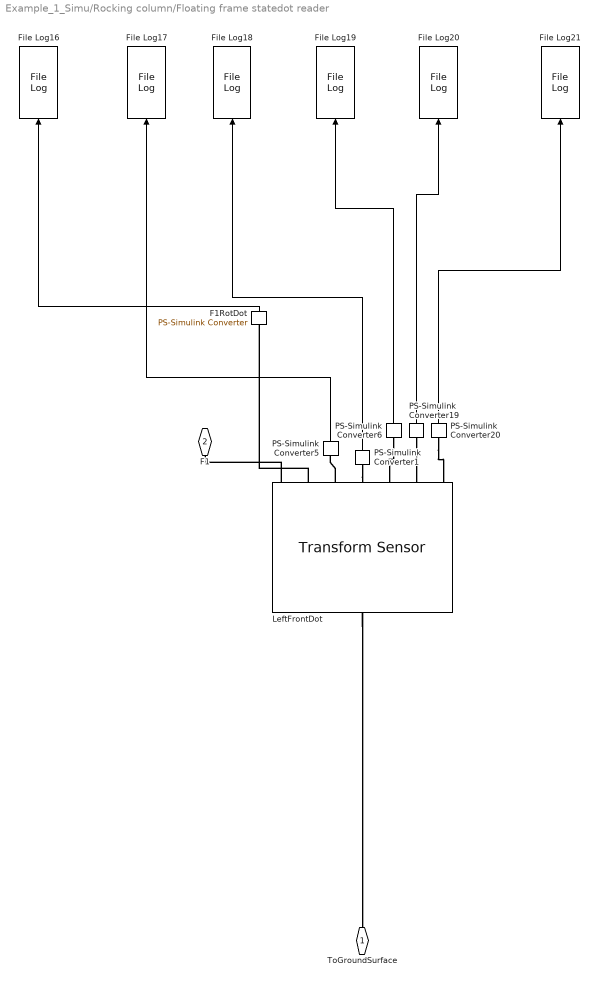
== system Example_1_Simu/Rocking column/Floating frame statedot reader ==
  " LeftFrontDot" : sm_lib/Frames and Transforms/Transform Sensor  MeasurementFrame=Base  RotationSequence=XYX  SenseAngle=off  SenseAxis=off  SenseQ=off  SenseR=off  SenseRotationSequence=off  SenseOmegaX=on  SenseOmegaY=on  SenseOmegaZ=on  SenseQDot=off  SenseRDot=off  SenseRotationSequenceDot=off  SenseAlphaX=off  SenseAlphaY=off  SenseAlphaZ=off  SenseQDDot=off  SenseRDDot=off  SenseX=off  SenseY=off  SenseZ=off  SenseRad=off  SenseAzim=off  SenseDist=off  SenseInc=off  SenseXDot=on  SenseYDot=on  SenseZDot=on  SenseRadDot=off  SenseAzimDot=off  SenseDistDot=off  SenseIncDot=off  SenseXDDot=off  SenseYDDot=off  SenseZDDot=off  SenseRadDDot=off  SenseAzimDDot=off  SenseDistDDot=off  SenseIncDDot=off
  F1RotDot : nesl_utility/PS-Simulink Converter  PhysicalDomain=network_engine_domain  SubClassName=ps_output  LeftPortType=input  RightPortType=output  PseudoPeriodic=off  Frequencies=[]  VectorFormat=1-D array  Unit=inherit  AffineConversion=off
  File Log{16,18..21} (5 alike) : slrealtimeloglib/File Log  decimation=200  inputProcessing=Elements as channels (sample based)
  File Log17 : slrealtimeloglib/File Log  decimation=10  inputProcessing=Elements as channels (sample based)
  PS-Simulink Converter{1,5..6,19..20} (5 alike) : nesl_utility/PS-Simulink Converter  PhysicalDomain=network_engine_domain  SubClassName=ps_output  LeftPortType=input  RightPortType=output  PseudoPeriodic=off  Frequencies=[]  VectorFormat=1-D array  Unit=inherit  AffineConversion=off
  ToGroundSurface : PMIOPort  Side=Left
  F1 : PMIOPort  Port=2  Side=Right
  wires:
  F1RotDot/1 -> File Log16/1
  PS-Simulink Converter5/1 -> File Log17/1
  PS-Simulink Converter1/1 -> File Log18/1
  PS-Simulink Converter6/1 -> File Log19/1
  PS-Simulink Converter19/1 -> File Log20/1
  PS-Simulink Converter20/1 -> File Log21/1
  connections:
  " LeftFrontDot"/LConn1 -- ToGroundSurface/RConn1
  " LeftFrontDot"/RConn2 -- F1RotDot/LConn1
  " LeftFrontDot"/RConn1 -- F1/RConn1
  " LeftFrontDot"/RConn3 -- PS-Simulink Converter5/LConn1
  PS-Simulink Converter1/LConn1 -- " LeftFrontDot"/RConn4
  PS-Simulink Converter6/LConn1 -- " LeftFrontDot"/RConn5
  PS-Simulink Converter19/LConn1 -- " LeftFrontDot"/RConn6
  PS-Simulink Converter20/LConn1 -- " LeftFrontDot"/RConn7
